simulink model "Model_14Bus_AC_DC_Microgrid"  (R2025a)
settings: Solver=ode23tb  StartTime=0.0  StopTime=0.1  MaxStep=1e-2  RelTol=1e-3
InitFcn:
  | Set_parameters_R2018
StopFcn:
  | Save_Data;
  | Graphics;
undefined symbols (not defined in the file): Clink, D1, Delta, dis1, dis10, dis11, dis12, dis13, dis14, dis2, dis3, dis4, dis5, dis6, dis7, dis8, dis9, Fc, Fnom, Hydride, Increment_MPPT, Ion, Ki_Ireg, Ki_VDCreg, Kp_Ireg, Kp_VDCreg, LimitL_Ireg, LimitL_VDCreg, Limits_MPPT, LimitU_Ireg, LimitU_VDCreg, Lithium, max_min, Metal, Nickel, P_Load_2, P_Load_3, Pnom, Pnom_T1, Pnom_T2, Pnom_T3, Pnom_xfo, Ql_Load_2, Ql_Load_3, R_Load_9, R_Load_DC, RL, Rl, RLff, Rls, sigbuilder_block, Ts, Ts_Control, Ts_Power, V1_LL_T3, Vf, Vfd, Vnom_dc, Vnom_DC, Vnom_Diesel ... (+5)
libraries: spsRMSLib x87, spsCurrentMeasurementLib x47, spsThreePhaseVIMeasurementLib x23, spsVoltageMeasurementLib x21, spsPowerLib x21, spsTHDLib x20, spsThreePhaseSeriesRLCBranchLib x20, spsSeriesRLCBranchLib x19, spsIGBTDiodeLib x14, spsThreePhaseBreakerLib x14, powerlib_extras x14, simulink x12
(part 5 of 9)

== system Model_14Bus_AC_DC_Microgrid/Boost -buck Bi-directional converter DC //CD 1 0.65 kW/ref ==
  note: 1 -charge
      | 0-discharge
  Constant2 : Constant  Value=max_min
  Constant3 : Constant  Value=max_min
  Current reference (battery charge) OP_Max : Constant  Value=5
  Current reference (battery discharge) OP_Max1 : Constant  Value=-5
  Min Demand OP_min : Constant  Value=3
  Min Demand OP_min1 : Constant  Value=-3
  Switch : Switch  Criteria=u2 > Threshold  SaturateOnIntegerOverflow=off  InputSameDT=off
  Switch1 : Switch  Criteria=u2 > Threshold  SaturateOnIntegerOverflow=off  InputSameDT=off
  Switch3 : Switch  Criteria=u2 > Threshold  SaturateOnIntegerOverflow=off  InputSameDT=off
  Vref1 : Constant
  ref : Outport  VectorParamsAs1DForOutWhenUnconnected=off
  wires:
  Constant3/1 -> Switch3/2
  Switch3/1 -> Switch/3
  Switch1/1 -> Switch/1
  Vref1/1 -> Switch/2
  Min Demand OP_min/1 -> Switch1/3
  Current reference (battery charge) OP_Max/1 -> Switch1/1
  Min Demand OP_min1/1 -> Switch3/3
  Constant2/1 -> Switch1/2
  Current reference (battery discharge) OP_Max1/1 -> Switch3/1
  Switch/1 -> ref/1

== system Model_14Bus_AC_DC_Microgrid/Boost converter DC //CD 2 5 kHz - 300V /  ==
  V_PV : Inport
  I_PV : Inport  Port=2
  Duty Cycle : Constant  Value=0.34
  PWM Generator (DC-DC) : spsPWMGeneratorDCDCLib/PWM Generator (DC-DC)  Fsw=fc  Ts=Ts_Power
  Terminator1 : Terminator
  Terminator2 : Terminator
  Pulses : Outport  VectorParamsAs1DForOutWhenUnconnected=off
  tag scope: D=global
  wires:
  V_PV/1 -> Terminator1/1
  I_PV/1 -> Terminator2/1
  PWM Generator (DC-DC)/1 -> Pulses/1
  Duty Cycle/1 -> [D], PWM Generator (DC-DC)/1

== system Model_14Bus_AC_DC_Microgrid/Bus_1/PLL ==
  Vabc_LN_pu : Inport
  2pi60'1 : Constant  Value=2*pi*60
  2pi60'2 : Constant  Value=2*pi*60
  2pi60'3 : Constant  Value=2*pi*60
  Constant : Constant  Value=90
  Demux : Demux  Outputs=3
  Gain1 : Gain  Gain=180/pi  SaturateOnIntegerOverflow=on  OutDataTypeStr=Inherit: Same as input  ParamDataTypeStr=Inherit: Same as input
  Gain2 : Gain  Gain=180/pi  SaturateOnIntegerOverflow=on  OutDataTypeStr=Inherit: Same as input  ParamDataTypeStr=Inherit: Same as input
  Gain3 : Gain  Gain=180/pi  SaturateOnIntegerOverflow=on  OutDataTypeStr=Inherit: Same as input  ParamDataTypeStr=Inherit: Same as input
  Mux : Mux  Inputs=3
  Pll1 : Subsystem
  Pll2 : Subsystem
  Pll3 : Subsystem
  Sum : Sum  Inputs=|++
  delta_abc : Outport  VectorParamsAs1DForOutWhenUnconnected=off
  wires:
  Vabc_LN_pu/1 -> Demux/1
  Demux/1 -> Pll3/1(señal)
  2pi60'3/1 -> Pll3/2(w)
  Pll3/1(f cos (rad)) -> Gain1/1
  Demux/2 -> Pll1/1(señal)
  2pi60'1/1 -> Pll1/2(w)
  Gain2/1 -> Mux/2
  Demux/3 -> Pll2/1(señal)
  2pi60'2/1 -> Pll2/2(w)
  Pll2/1(f cos (rad)) -> Gain3/1
  Gain3/1 -> Mux/3
  Pll1/1(f cos (rad)) -> Gain2/1
  Mux/1 -> Sum/1
  Gain1/1 -> Mux/1
  Constant/1 -> Sum/2
  Sum/1 -> delta_abc/1

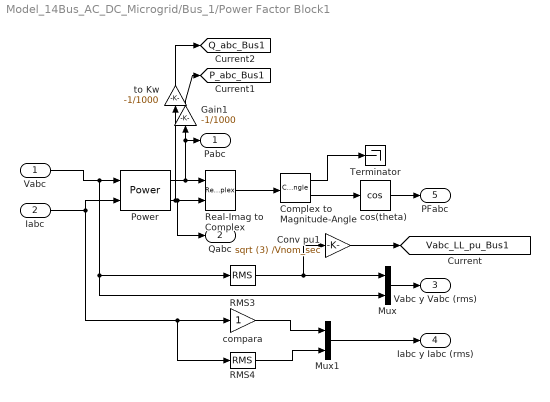
== system Model_14Bus_AC_DC_Microgrid/Bus_1/Power Factor Block1 ==
  Vabc : Inport
  Iabc : Inport  Port=2
  Complex to Magnitude-Angle : ComplexToMagnitudeAngle
  Conv pu1 : Gain  Gain=sqrt (3) /Vnom_sec  SaturateOnIntegerOverflow=on  OutDataTypeStr=Inherit: Same as input  ParamDataTypeStr=Inherit: Same as input
  Gain1 : Gain  Gain=-1/1000
  Mux : Mux  Inputs=2
  Mux1 : Mux  Inputs=2
  Power : spsPowerLib/Power  Freq=Freq  Vinit=Vinit  Iinit=Iinit  Ts=Ts
  RMS3 : spsRMSLib/RMS  TrueRMS=on  Freq=60  RMSInit=0  Ts=0
  RMS4 : spsRMSLib/RMS  TrueRMS=on  Freq=60  RMSInit=0  Ts=0
  Real-Imag to Complex : RealImagToComplex
  Terminator : Terminator
  compara : Gain  SaturateOnIntegerOverflow=on  OutDataTypeStr=Inherit: Same as input  ParamDataTypeStr=Inherit: Same as input
  cos(theta) : Trigonometry  Operator=cos
  to Kw : Gain  Gain=-1/1000
  Pabc : Outport  VectorParamsAs1DForOutWhenUnconnected=off
  Qabc : Outport  Port=2  VectorParamsAs1DForOutWhenUnconnected=off
  Vabc y Vabc (rms) : Outport  Port=3  VectorParamsAs1DForOutWhenUnconnected=off
  Iabc y Iabc (rms) : Outport  Port=4  VectorParamsAs1DForOutWhenUnconnected=off
  "PFabc " : Outport  Port=5  VectorParamsAs1DForOutWhenUnconnected=off
  tag scope: P_abc_Bus1=global, Q_abc_Bus1=global, Vabc_LL_pu_Bus1=global
  wires:
  Power/1 -> Gain1/1, Pabc/1, Real-Imag to Complex/1
  Power/2 -> Qabc/1, Real-Imag to Complex/2, to Kw/1
  Complex to Magnitude-Angle/2 -> cos(theta)/1
  Real-Imag to Complex/1 -> Complex to Magnitude-Angle/1
  cos(theta)/1 -> "PFabc "/1
  Complex to Magnitude-Angle/1 -> Terminator/1
  Iabc/1 -> RMS4/1, compara/1, Power/2
  RMS4/1 -> Mux1/2
  Mux1/1 -> Iabc y Iabc (rms)/1
  Mux/1 -> Vabc y Vabc (rms)/1
  Vabc/1 -> Power/1, Mux/2, RMS3/1
  compara/1 -> Mux1/1
  RMS3/1 -> Conv pu1/1, Mux/1
  Conv pu1/1 -> [Vabc_LL_pu_Bus1]
  to Kw/1 -> [Q_abc_Bus1]
  Gain1/1 -> [P_abc_Bus1]

== system Model_14Bus_AC_DC_Microgrid/Bus_10/PLL ==
  Vabc_LN_pu : Inport
  2pi60'1 : Constant  Value=2*pi*60
  2pi60'2 : Constant  Value=2*pi*60
  2pi60'3 : Constant  Value=2*pi*60
  Constant : Constant  Value=90
  Demux : Demux  Outputs=3
  Gain1 : Gain  Gain=180/pi  SaturateOnIntegerOverflow=on  OutDataTypeStr=Inherit: Same as input  ParamDataTypeStr=Inherit: Same as input
  Gain2 : Gain  Gain=180/pi  SaturateOnIntegerOverflow=on  OutDataTypeStr=Inherit: Same as input  ParamDataTypeStr=Inherit: Same as input
  Gain3 : Gain  Gain=180/pi  SaturateOnIntegerOverflow=on  OutDataTypeStr=Inherit: Same as input  ParamDataTypeStr=Inherit: Same as input
  Mux : Mux  Inputs=3
  Pll1 : Subsystem
  Pll2 : Subsystem
  Pll3 : Subsystem
  Sum : Sum  Inputs=|++
  delta_abc : Outport  VectorParamsAs1DForOutWhenUnconnected=off
  wires:
  Vabc_LN_pu/1 -> Demux/1
  Demux/1 -> Pll3/1(señal)
  2pi60'3/1 -> Pll3/2(w)
  Pll3/1(f cos (rad)) -> Gain1/1
  Demux/2 -> Pll1/1(señal)
  2pi60'1/1 -> Pll1/2(w)
  Gain2/1 -> Mux/2
  Demux/3 -> Pll2/1(señal)
  2pi60'2/1 -> Pll2/2(w)
  Pll2/1(f cos (rad)) -> Gain3/1
  Gain3/1 -> Mux/3
  Pll1/1(f cos (rad)) -> Gain2/1
  Mux/1 -> Sum/1
  Gain1/1 -> Mux/1
  Constant/1 -> Sum/2
  Sum/1 -> delta_abc/1

== system Model_14Bus_AC_DC_Microgrid/Bus_10/Power Factor Block1 ==
  Vabc : Inport
  Iabc : Inport  Port=2
  Complex to Magnitude-Angle : ComplexToMagnitudeAngle
  Conv pu2 : Gain  Gain=sqrt (3) /Vnom_prim  SaturateOnIntegerOverflow=on  OutDataTypeStr=Inherit: Same as input  ParamDataTypeStr=Inherit: Same as input
  Mux : Mux  Inputs=2
  Mux1 : Mux  Inputs=2
  Power : spsPowerLib/Power  Freq=Freq  Vinit=Vinit  Iinit=Iinit  Ts=Ts
  RMS3 : spsRMSLib/RMS  TrueRMS=on  Freq=60  RMSInit=0  Ts=0
  RMS4 : spsRMSLib/RMS  TrueRMS=on  Freq=60  RMSInit=0  Ts=0
  Real-Imag to Complex : RealImagToComplex
  Terminator : Terminator
  compara : Gain  SaturateOnIntegerOverflow=on  OutDataTypeStr=Inherit: Same as input  ParamDataTypeStr=Inherit: Same as input
  cos(theta) : Trigonometry  Operator=cos
  to Kw : Gain  Gain=1/1000
  to Kw1 : Gain  Gain=1/1000
  Pabc : Outport  VectorParamsAs1DForOutWhenUnconnected=off
  Qabc : Outport  Port=2  VectorParamsAs1DForOutWhenUnconnected=off
  Vabc y Vabc (rms) : Outport  Port=3  VectorParamsAs1DForOutWhenUnconnected=off
  Iabc y Iabc (rms) : Outport  Port=4  VectorParamsAs1DForOutWhenUnconnected=off
  "PFabc " : Outport  Port=5  VectorParamsAs1DForOutWhenUnconnected=off
  tag scope: P_abc_Bus10=global, Q_abc_Bus10=global, Vabc_LL_pu_Bus10=global
  wires:
  Complex to Magnitude-Angle/2 -> cos(theta)/1
  Real-Imag to Complex/1 -> Complex to Magnitude-Angle/1
  cos(theta)/1 -> "PFabc "/1
  Complex to Magnitude-Angle/1 -> Terminator/1
  Iabc/1 -> RMS4/1, compara/1, Power/2
  RMS4/1 -> Mux1/2
  Mux1/1 -> Iabc y Iabc (rms)/1
  Mux/1 -> Vabc y Vabc (rms)/1
  Vabc/1 -> Power/1, Mux/2, RMS3/1
  compara/1 -> Mux1/1
  Conv pu2/1 -> [Vabc_LL_pu_Bus10]
  RMS3/1 -> Conv pu2/1, Mux/1
  Power/1 -> to Kw1/1, Pabc/1, Real-Imag to Complex/1
  Power/2 -> Qabc/1, Real-Imag to Complex/2, to Kw/1
  to Kw/1 -> [Q_abc_Bus10]
  to Kw1/1 -> [P_abc_Bus10]

== system Model_14Bus_AC_DC_Microgrid/Bus_11/PLL ==
  Vabc_LN_pu : Inport
  2pi60'1 : Constant  Value=2*pi*60
  2pi60'2 : Constant  Value=2*pi*60
  2pi60'3 : Constant  Value=2*pi*60
  Constant : Constant  Value=90
  Demux : Demux  Outputs=3
  Gain1 : Gain  Gain=180/pi  SaturateOnIntegerOverflow=on  OutDataTypeStr=Inherit: Same as input  ParamDataTypeStr=Inherit: Same as input
  Gain2 : Gain  Gain=180/pi  SaturateOnIntegerOverflow=on  OutDataTypeStr=Inherit: Same as input  ParamDataTypeStr=Inherit: Same as input
  Gain3 : Gain  Gain=180/pi  SaturateOnIntegerOverflow=on  OutDataTypeStr=Inherit: Same as input  ParamDataTypeStr=Inherit: Same as input
  Mux : Mux  Inputs=3
  Pll1 : Subsystem
  Pll2 : Subsystem
  Pll3 : Subsystem
  Sum : Sum  Inputs=|++
  delta_abc : Outport  VectorParamsAs1DForOutWhenUnconnected=off
  wires:
  Vabc_LN_pu/1 -> Demux/1
  Demux/1 -> Pll3/1(señal)
  2pi60'3/1 -> Pll3/2(w)
  Pll3/1(f cos (rad)) -> Gain1/1
  Demux/2 -> Pll1/1(señal)
  2pi60'1/1 -> Pll1/2(w)
  Gain2/1 -> Mux/2
  Demux/3 -> Pll2/1(señal)
  2pi60'2/1 -> Pll2/2(w)
  Pll2/1(f cos (rad)) -> Gain3/1
  Gain3/1 -> Mux/3
  Pll1/1(f cos (rad)) -> Gain2/1
  Mux/1 -> Sum/1
  Gain1/1 -> Mux/1
  Constant/1 -> Sum/2
  Sum/1 -> delta_abc/1

== system Model_14Bus_AC_DC_Microgrid/Bus_11/Power Factor Block1 ==
  Vabc : Inport
  Iabc : Inport  Port=2
  Complex to Magnitude-Angle : ComplexToMagnitudeAngle
  Conv pu2 : Gain  Gain=sqrt (3) /Vnom_prim  SaturateOnIntegerOverflow=on  OutDataTypeStr=Inherit: Same as input  ParamDataTypeStr=Inherit: Same as input
  Mux : Mux  Inputs=2
  Mux1 : Mux  Inputs=2
  Power : spsPowerLib/Power  Freq=Freq  Vinit=Vinit  Iinit=Iinit  Ts=Ts
  RMS3 : spsRMSLib/RMS  TrueRMS=on  Freq=60  RMSInit=0  Ts=0
  RMS4 : spsRMSLib/RMS  TrueRMS=on  Freq=60  RMSInit=0  Ts=0
  Real-Imag to Complex : RealImagToComplex
  Terminator : Terminator
  compara : Gain  SaturateOnIntegerOverflow=on  OutDataTypeStr=Inherit: Same as input  ParamDataTypeStr=Inherit: Same as input
  cos(theta) : Trigonometry  Operator=cos
  to Kw : Gain  Gain=1/1000
  to Kw1 : Gain  Gain=1/1000
  Pabc : Outport  VectorParamsAs1DForOutWhenUnconnected=off
  Qabc : Outport  Port=2  VectorParamsAs1DForOutWhenUnconnected=off
  Vabc y Vabc (rms) : Outport  Port=3  VectorParamsAs1DForOutWhenUnconnected=off
  Iabc y Iabc (rms) : Outport  Port=4  VectorParamsAs1DForOutWhenUnconnected=off
  "PFabc " : Outport  Port=5  VectorParamsAs1DForOutWhenUnconnected=off
  tag scope: P_abc_Bus11=global, Q_abc_Bus11=global, Vabc_LL_pu_Bus11=global
  wires:
  Complex to Magnitude-Angle/2 -> cos(theta)/1
  Real-Imag to Complex/1 -> Complex to Magnitude-Angle/1
  cos(theta)/1 -> "PFabc "/1
  Complex to Magnitude-Angle/1 -> Terminator/1
  Iabc/1 -> RMS4/1, compara/1, Power/2
  RMS4/1 -> Mux1/2
  Mux1/1 -> Iabc y Iabc (rms)/1
  Mux/1 -> Vabc y Vabc (rms)/1
  Vabc/1 -> Power/1, Mux/2, RMS3/1
  compara/1 -> Mux1/1
  RMS3/1 -> Conv pu2/1, Mux/1
  Conv pu2/1 -> [Vabc_LL_pu_Bus11]
  Power/2 -> Qabc/1, Real-Imag to Complex/2, to Kw/1
  Power/1 -> to Kw1/1, Pabc/1, Real-Imag to Complex/1
  to Kw/1 -> [Q_abc_Bus11]
  to Kw1/1 -> [P_abc_Bus11]

== system Model_14Bus_AC_DC_Microgrid/Bus_12/PLL ==
  Vabc_LN_pu : Inport
  2pi60'1 : Constant  Value=2*pi*60
  2pi60'2 : Constant  Value=2*pi*60
  2pi60'3 : Constant  Value=2*pi*60
  Constant : Constant  Value=90
  Demux : Demux  Outputs=3
  Gain1 : Gain  Gain=180/pi  SaturateOnIntegerOverflow=on  OutDataTypeStr=Inherit: Same as input  ParamDataTypeStr=Inherit: Same as input
  Gain2 : Gain  Gain=180/pi  SaturateOnIntegerOverflow=on  OutDataTypeStr=Inherit: Same as input  ParamDataTypeStr=Inherit: Same as input
  Gain3 : Gain  Gain=180/pi  SaturateOnIntegerOverflow=on  OutDataTypeStr=Inherit: Same as input  ParamDataTypeStr=Inherit: Same as input
  Mux : Mux  Inputs=3
  Pll1 : Subsystem
  Pll2 : Subsystem
  Pll3 : Subsystem
  Sum : Sum  Inputs=|++
  delta_abc : Outport  VectorParamsAs1DForOutWhenUnconnected=off
  wires:
  Vabc_LN_pu/1 -> Demux/1
  Demux/1 -> Pll3/1(señal)
  2pi60'3/1 -> Pll3/2(w)
  Pll3/1(f cos (rad)) -> Gain1/1
  Demux/2 -> Pll1/1(señal)
  2pi60'1/1 -> Pll1/2(w)
  Gain2/1 -> Mux/2
  Demux/3 -> Pll2/1(señal)
  2pi60'2/1 -> Pll2/2(w)
  Pll2/1(f cos (rad)) -> Gain3/1
  Gain3/1 -> Mux/3
  Pll1/1(f cos (rad)) -> Gain2/1
  Mux/1 -> Sum/1
  Gain1/1 -> Mux/1
  Constant/1 -> Sum/2
  Sum/1 -> delta_abc/1

== system Model_14Bus_AC_DC_Microgrid/Bus_12/Power Factor Block1 ==
  Vabc : Inport
  Iabc : Inport  Port=2
  Complex to Magnitude-Angle : ComplexToMagnitudeAngle
  Conv pu2 : Gain  Gain=sqrt (3) /Vnom_prim  SaturateOnIntegerOverflow=on  OutDataTypeStr=Inherit: Same as input  ParamDataTypeStr=Inherit: Same as input
  Mux : Mux  Inputs=2
  Mux1 : Mux  Inputs=2
  Power : spsPowerLib/Power  Freq=Freq  Vinit=Vinit  Iinit=Iinit  Ts=Ts
  RMS3 : spsRMSLib/RMS  TrueRMS=on  Freq=60  RMSInit=0  Ts=0
  RMS4 : spsRMSLib/RMS  TrueRMS=on  Freq=60  RMSInit=0  Ts=0
  Real-Imag to Complex : RealImagToComplex
  Terminator : Terminator
  compara : Gain  SaturateOnIntegerOverflow=on  OutDataTypeStr=Inherit: Same as input  ParamDataTypeStr=Inherit: Same as input
  cos(theta) : Trigonometry  Operator=cos
  to Kw : Gain  Gain=1/1000
  to Kw1 : Gain  Gain=1/1000
  Pabc : Outport  VectorParamsAs1DForOutWhenUnconnected=off
  Qabc : Outport  Port=2  VectorParamsAs1DForOutWhenUnconnected=off
  Vabc y Vabc (rms) : Outport  Port=3  VectorParamsAs1DForOutWhenUnconnected=off
  Iabc y Iabc (rms) : Outport  Port=4  VectorParamsAs1DForOutWhenUnconnected=off
  "PFabc " : Outport  Port=5  VectorParamsAs1DForOutWhenUnconnected=off
  tag scope: P_abc_Bus12=global, Q_abc_Bus12=global, Vabc_LL_pu_Bus12=global
  wires:
  Complex to Magnitude-Angle/2 -> cos(theta)/1
  Real-Imag to Complex/1 -> Complex to Magnitude-Angle/1
  cos(theta)/1 -> "PFabc "/1
  Complex to Magnitude-Angle/1 -> Terminator/1
  Iabc/1 -> RMS4/1, compara/1, Power/2
  RMS4/1 -> Mux1/2
  Mux1/1 -> Iabc y Iabc (rms)/1
  Mux/1 -> Vabc y Vabc (rms)/1
  Vabc/1 -> Power/1, Mux/2, RMS3/1
  compara/1 -> Mux1/1
  RMS3/1 -> Conv pu2/1, Mux/1
  Conv pu2/1 -> [Vabc_LL_pu_Bus12]
  Power/1 -> to Kw/1, Pabc/1, Real-Imag to Complex/1
  Power/2 -> to Kw1/1, Qabc/1, Real-Imag to Complex/2
  to Kw1/1 -> [Q_abc_Bus12]
  to Kw/1 -> [P_abc_Bus12]

== system Model_14Bus_AC_DC_Microgrid/Bus_14 /PLL ==
  Vabc_LN_pu : Inport
  2pi60'1 : Constant  Value=2*pi*60
  2pi60'2 : Constant  Value=2*pi*60
  2pi60'3 : Constant  Value=2*pi*60
  Constant : Constant  Value=90
  Demux : Demux  Outputs=3
  Gain1 : Gain  Gain=180/pi  SaturateOnIntegerOverflow=on  OutDataTypeStr=Inherit: Same as input  ParamDataTypeStr=Inherit: Same as input
  Gain2 : Gain  Gain=180/pi  SaturateOnIntegerOverflow=on  OutDataTypeStr=Inherit: Same as input  ParamDataTypeStr=Inherit: Same as input
  Gain3 : Gain  Gain=180/pi  SaturateOnIntegerOverflow=on  OutDataTypeStr=Inherit: Same as input  ParamDataTypeStr=Inherit: Same as input
  Mux : Mux  Inputs=3
  Pll1 : Subsystem
  Pll2 : Subsystem
  Pll3 : Subsystem
  Sum : Sum  Inputs=|++
  delta_abc : Outport  VectorParamsAs1DForOutWhenUnconnected=off
  wires:
  Vabc_LN_pu/1 -> Demux/1
  Demux/1 -> Pll3/1(señal)
  2pi60'3/1 -> Pll3/2(w)
  Pll3/1(f cos (rad)) -> Gain1/1
  Demux/2 -> Pll1/1(señal)
  2pi60'1/1 -> Pll1/2(w)
  Gain2/1 -> Mux/2
  Demux/3 -> Pll2/1(señal)
  2pi60'2/1 -> Pll2/2(w)
  Pll2/1(f cos (rad)) -> Gain3/1
  Gain3/1 -> Mux/3
  Pll1/1(f cos (rad)) -> Gain2/1
  Mux/1 -> Sum/1
  Gain1/1 -> Mux/1
  Constant/1 -> Sum/2
  Sum/1 -> delta_abc/1

== system Model_14Bus_AC_DC_Microgrid/Bus_14 /Power Factor Block1 ==
  Vabc : Inport
  Iabc : Inport  Port=2
  Complex to Magnitude-Angle : ComplexToMagnitudeAngle
  Conv pu2 : Gain  Gain=sqrt (3) /Vnom_prim  SaturateOnIntegerOverflow=on  OutDataTypeStr=Inherit: Same as input  ParamDataTypeStr=Inherit: Same as input
  Mux : Mux  Inputs=2
  Mux1 : Mux  Inputs=2
  Power : spsPowerLib/Power  Freq=Freq  Vinit=Vinit  Iinit=Iinit  Ts=Ts
  RMS3 : spsRMSLib/RMS  TrueRMS=on  Freq=60  RMSInit=0  Ts=0
  RMS4 : spsRMSLib/RMS  TrueRMS=on  Freq=60  RMSInit=0  Ts=0
  Real-Imag to Complex : RealImagToComplex
  Terminator : Terminator
  compara : Gain  SaturateOnIntegerOverflow=on  OutDataTypeStr=Inherit: Same as input  ParamDataTypeStr=Inherit: Same as input
  cos(theta) : Trigonometry  Operator=cos
  to Kw : Gain  Gain=1/1000
  to Kw1 : Gain  Gain=1/1000
  Pabc : Outport  VectorParamsAs1DForOutWhenUnconnected=off
  Qabc : Outport  Port=2  VectorParamsAs1DForOutWhenUnconnected=off
  Vabc y Vabc (rms) : Outport  Port=3  VectorParamsAs1DForOutWhenUnconnected=off
  Iabc y Iabc (rms) : Outport  Port=4  VectorParamsAs1DForOutWhenUnconnected=off
  "PFabc " : Outport  Port=5  VectorParamsAs1DForOutWhenUnconnected=off
  tag scope: P_abc_Bus14=global, Q_abc_Bus14=global, Vabc_LL_pu_Bus14=global
  wires:
  Complex to Magnitude-Angle/2 -> cos(theta)/1
  Real-Imag to Complex/1 -> Complex to Magnitude-Angle/1
  cos(theta)/1 -> "PFabc "/1
  Complex to Magnitude-Angle/1 -> Terminator/1
  Iabc/1 -> RMS4/1, compara/1, Power/2
  RMS4/1 -> Mux1/2
  Mux1/1 -> Iabc y Iabc (rms)/1
  Mux/1 -> Vabc y Vabc (rms)/1
  Vabc/1 -> Power/1, Mux/2, RMS3/1
  compara/1 -> Mux1/1
  RMS3/1 -> Conv pu2/1, Mux/1
  Conv pu2/1 -> [Vabc_LL_pu_Bus14]
  Power/2 -> Qabc/1, Real-Imag to Complex/2, to Kw1/1
  Power/1 -> to Kw/1, Pabc/1, Real-Imag to Complex/1
  to Kw1/1 -> [Q_abc_Bus14]
  to Kw/1 -> [P_abc_Bus14]

== system Model_14Bus_AC_DC_Microgrid/Bus_2/PLL ==
  Vabc_LN_pu : Inport
  2pi60'1 : Constant  Value=2*pi*60
  2pi60'2 : Constant  Value=2*pi*60
  2pi60'3 : Constant  Value=2*pi*60
  Constant : Constant  Value=90
  Demux : Demux  Outputs=3
  Gain1 : Gain  Gain=180/pi  SaturateOnIntegerOverflow=on  OutDataTypeStr=Inherit: Same as input  ParamDataTypeStr=Inherit: Same as input
  Gain2 : Gain  Gain=180/pi  SaturateOnIntegerOverflow=on  OutDataTypeStr=Inherit: Same as input  ParamDataTypeStr=Inherit: Same as input
  Gain3 : Gain  Gain=180/pi  SaturateOnIntegerOverflow=on  OutDataTypeStr=Inherit: Same as input  ParamDataTypeStr=Inherit: Same as input
  Mux : Mux  Inputs=3
  Pll1 : Subsystem
  Pll2 : Subsystem
  Pll3 : Subsystem
  Sum : Sum  Inputs=|++
  delta_abc : Outport  VectorParamsAs1DForOutWhenUnconnected=off
  wires:
  Vabc_LN_pu/1 -> Demux/1
  Demux/1 -> Pll3/1(señal)
  2pi60'3/1 -> Pll3/2(w)
  Pll3/1(f cos (rad)) -> Gain1/1
  Demux/2 -> Pll1/1(señal)
  2pi60'1/1 -> Pll1/2(w)
  Gain2/1 -> Mux/2
  Demux/3 -> Pll2/1(señal)
  2pi60'2/1 -> Pll2/2(w)
  Pll2/1(f cos (rad)) -> Gain3/1
  Gain3/1 -> Mux/3
  Pll1/1(f cos (rad)) -> Gain2/1
  Mux/1 -> Sum/1
  Gain1/1 -> Mux/1
  Constant/1 -> Sum/2
  Sum/1 -> delta_abc/1

== system Model_14Bus_AC_DC_Microgrid/Bus_2/Power Factor Block1 ==
  Vabc : Inport
  Iabc : Inport  Port=2
  Complex to Magnitude-Angle : ComplexToMagnitudeAngle
  Conv pu1 : Gain  Gain=sqrt (3) /Vnom_sec  SaturateOnIntegerOverflow=on  OutDataTypeStr=Inherit: Same as input  ParamDataTypeStr=Inherit: Same as input
  Mux : Mux  Inputs=2
  Mux1 : Mux  Inputs=2
  Power : spsPowerLib/Power  Freq=Freq  Vinit=Vinit  Iinit=Iinit  Ts=Ts
  RMS3 : spsRMSLib/RMS  TrueRMS=on  Freq=60  RMSInit=0  Ts=0
  RMS4 : spsRMSLib/RMS  TrueRMS=on  Freq=60  RMSInit=0  Ts=0
  Real-Imag to Complex : RealImagToComplex
  Terminator : Terminator
  compara : Gain  SaturateOnIntegerOverflow=on  OutDataTypeStr=Inherit: Same as input  ParamDataTypeStr=Inherit: Same as input
  cos(theta) : Trigonometry  Operator=cos
  to Kw : Gain  Gain=-1/1000
  to Kw1 : Gain  Gain=-1/1000
  Pabc : Outport  VectorParamsAs1DForOutWhenUnconnected=off
  Qabc : Outport  Port=2  VectorParamsAs1DForOutWhenUnconnected=off
  Vabc y Vabc (rms) : Outport  Port=3  VectorParamsAs1DForOutWhenUnconnected=off
  Iabc y Iabc (rms) : Outport  Port=4  VectorParamsAs1DForOutWhenUnconnected=off
  "PFabc " : Outport  Port=5  VectorParamsAs1DForOutWhenUnconnected=off
  tag scope: P_abc_Bus2=global, Q_abc_Bus2=global, Vabc_LL_pu_Bus2=global
  wires:
  Complex to Magnitude-Angle/2 -> cos(theta)/1
  Real-Imag to Complex/1 -> Complex to Magnitude-Angle/1
  cos(theta)/1 -> "PFabc "/1
  Complex to Magnitude-Angle/1 -> Terminator/1
  Iabc/1 -> RMS4/1, compara/1, Power/2
  RMS4/1 -> Mux1/2
  Mux1/1 -> Iabc y Iabc (rms)/1
  Mux/1 -> Vabc y Vabc (rms)/1
  Vabc/1 -> Power/1, Mux/2, RMS3/1
  compara/1 -> Mux1/1
  RMS3/1 -> Conv pu1/1, Mux/1
  Conv pu1/1 -> [Vabc_LL_pu_Bus2]
  Power/1 -> to Kw1/1, Pabc/1, Real-Imag to Complex/1
  Power/2 -> to Kw/1, Qabc/1, Real-Imag to Complex/2
  to Kw/1 -> [Q_abc_Bus2]
  to Kw1/1 -> [P_abc_Bus2]

== system Model_14Bus_AC_DC_Microgrid/Bus_3/PLL ==
  Vabc_LN_pu : Inport
  2pi60'1 : Constant  Value=2*pi*60
  2pi60'2 : Constant  Value=2*pi*60
  2pi60'3 : Constant  Value=2*pi*60
  Constant : Constant  Value=90
  Demux : Demux  Outputs=3
  Gain1 : Gain  Gain=180/pi  SaturateOnIntegerOverflow=on  OutDataTypeStr=Inherit: Same as input  ParamDataTypeStr=Inherit: Same as input
  Gain2 : Gain  Gain=180/pi  SaturateOnIntegerOverflow=on  OutDataTypeStr=Inherit: Same as input  ParamDataTypeStr=Inherit: Same as input
  Gain3 : Gain  Gain=180/pi  SaturateOnIntegerOverflow=on  OutDataTypeStr=Inherit: Same as input  ParamDataTypeStr=Inherit: Same as input
  Mux : Mux  Inputs=3
  Pll1 : Subsystem
  Pll2 : Subsystem
  Pll3 : Subsystem
  Sum : Sum  Inputs=|++
  delta_abc : Outport  VectorParamsAs1DForOutWhenUnconnected=off
  wires:
  Vabc_LN_pu/1 -> Demux/1
  Demux/1 -> Pll3/1(señal)
  2pi60'3/1 -> Pll3/2(w)
  Pll3/1(f cos (rad)) -> Gain1/1
  Demux/2 -> Pll1/1(señal)
  2pi60'1/1 -> Pll1/2(w)
  Gain2/1 -> Mux/2
  Demux/3 -> Pll2/1(señal)
  2pi60'2/1 -> Pll2/2(w)
  Pll2/1(f cos (rad)) -> Gain3/1
  Gain3/1 -> Mux/3
  Pll1/1(f cos (rad)) -> Gain2/1
  Mux/1 -> Sum/1
  Gain1/1 -> Mux/1
  Constant/1 -> Sum/2
  Sum/1 -> delta_abc/1

== system Model_14Bus_AC_DC_Microgrid/Bus_3/Power Factor Block1 ==
  Vabc : Inport
  Iabc : Inport  Port=2
  Complex to Magnitude-Angle : ComplexToMagnitudeAngle
  Conv pu1 : Gain  Gain=sqrt (3) /Vnom_sec  SaturateOnIntegerOverflow=on  OutDataTypeStr=Inherit: Same as input  ParamDataTypeStr=Inherit: Same as input
  Mux : Mux  Inputs=2
  Mux1 : Mux  Inputs=2
  Power : spsPowerLib/Power  Freq=Freq  Vinit=Vinit  Iinit=Iinit  Ts=Ts
  RMS3 : spsRMSLib/RMS  TrueRMS=on  Freq=60  RMSInit=0  Ts=0
  RMS4 : spsRMSLib/RMS  TrueRMS=on  Freq=60  RMSInit=0  Ts=0
  Real-Imag to Complex : RealImagToComplex
  Terminator : Terminator
  compara : Gain  SaturateOnIntegerOverflow=on  OutDataTypeStr=Inherit: Same as input  ParamDataTypeStr=Inherit: Same as input
  cos(theta) : Trigonometry  Operator=cos
  to Kw : Gain  Gain=1/1000
  to Kw1 : Gain  Gain=1/1000
  Pabc : Outport  VectorParamsAs1DForOutWhenUnconnected=off
  Qabc : Outport  Port=2  VectorParamsAs1DForOutWhenUnconnected=off
  Vabc y Vabc (rms) : Outport  Port=3  VectorParamsAs1DForOutWhenUnconnected=off
  Iabc y Iabc (rms) : Outport  Port=4  VectorParamsAs1DForOutWhenUnconnected=off
  "PFabc " : Outport  Port=5  VectorParamsAs1DForOutWhenUnconnected=off
  tag scope: P_abc_Bus3=global, Q_abc_Bus3=global, Vabc_LL_pu_Bus3=global
  wires:
  Complex to Magnitude-Angle/2 -> cos(theta)/1
  Real-Imag to Complex/1 -> Complex to Magnitude-Angle/1
  cos(theta)/1 -> "PFabc "/1
  Complex to Magnitude-Angle/1 -> Terminator/1
  Iabc/1 -> RMS4/1, compara/1, Power/2
  RMS4/1 -> Mux1/2
  Mux1/1 -> Iabc y Iabc (rms)/1
  Mux/1 -> Vabc y Vabc (rms)/1
  Vabc/1 -> Power/1, Mux/2, RMS3/1
  compara/1 -> Mux1/1
  Conv pu1/1 -> [Vabc_LL_pu_Bus3]
  RMS3/1 -> Conv pu1/1, Mux/1
  Power/2 -> Qabc/1, Real-Imag to Complex/2, to Kw/1
  Power/1 -> to Kw1/1, Pabc/1, Real-Imag to Complex/1
  to Kw/1 -> [Q_abc_Bus3]
  to Kw1/1 -> [P_abc_Bus3]

== system Model_14Bus_AC_DC_Microgrid/Bus_4/PLL ==
  Vabc_LN_pu : Inport
  2pi60'1 : Constant  Value=2*pi*60
  2pi60'2 : Constant  Value=2*pi*60
  2pi60'3 : Constant  Value=2*pi*60
  Constant : Constant  Value=90
  Demux : Demux  Outputs=3
  Gain1 : Gain  Gain=180/pi  SaturateOnIntegerOverflow=on  OutDataTypeStr=Inherit: Same as input  ParamDataTypeStr=Inherit: Same as input
  Gain2 : Gain  Gain=180/pi  SaturateOnIntegerOverflow=on  OutDataTypeStr=Inherit: Same as input  ParamDataTypeStr=Inherit: Same as input
  Gain3 : Gain  Gain=180/pi  SaturateOnIntegerOverflow=on  OutDataTypeStr=Inherit: Same as input  ParamDataTypeStr=Inherit: Same as input
  Mux : Mux  Inputs=3
  Pll1 : Subsystem
  Pll2 : Subsystem
  Pll3 : Subsystem
  Sum : Sum  Inputs=|++
  delta_abc : Outport  VectorParamsAs1DForOutWhenUnconnected=off
  wires:
  Vabc_LN_pu/1 -> Demux/1
  Demux/1 -> Pll3/1(señal)
  2pi60'3/1 -> Pll3/2(w)
  Pll3/1(f cos (rad)) -> Gain1/1
  Demux/2 -> Pll1/1(señal)
  2pi60'1/1 -> Pll1/2(w)
  Gain2/1 -> Mux/2
  Demux/3 -> Pll2/1(señal)
  2pi60'2/1 -> Pll2/2(w)
  Pll2/1(f cos (rad)) -> Gain3/1
  Gain3/1 -> Mux/3
  Pll1/1(f cos (rad)) -> Gain2/1
  Mux/1 -> Sum/1
  Gain1/1 -> Mux/1
  Constant/1 -> Sum/2
  Sum/1 -> delta_abc/1

== system Model_14Bus_AC_DC_Microgrid/Bus_4/Power Factor Block1 ==
  Vabc : Inport
  Iabc : Inport  Port=2
  Complex to Magnitude-Angle : ComplexToMagnitudeAngle
  Conv pu1 : Gain  Gain=sqrt (3) /Vnom_sec  SaturateOnIntegerOverflow=on  OutDataTypeStr=Inherit: Same as input  ParamDataTypeStr=Inherit: Same as input
  Mux : Mux  Inputs=2
  Mux1 : Mux  Inputs=2
  Power : spsPowerLib/Power  Freq=Freq  Vinit=Vinit  Iinit=Iinit  Ts=Ts
  RMS3 : spsRMSLib/RMS  TrueRMS=on  Freq=60  RMSInit=0  Ts=0
  RMS4 : spsRMSLib/RMS  TrueRMS=on  Freq=60  RMSInit=0  Ts=0
  Real-Imag to Complex : RealImagToComplex
  Terminator : Terminator
  compara : Gain  SaturateOnIntegerOverflow=on  OutDataTypeStr=Inherit: Same as input  ParamDataTypeStr=Inherit: Same as input
  cos(theta) : Trigonometry  Operator=cos
  to Kw : Gain  Gain=1/1000
  to Kw1 : Gain  Gain=1/1000
  Pabc : Outport  VectorParamsAs1DForOutWhenUnconnected=off
  Qabc : Outport  Port=2  VectorParamsAs1DForOutWhenUnconnected=off
  Vabc y Vabc (rms) : Outport  Port=3  VectorParamsAs1DForOutWhenUnconnected=off
  Iabc y Iabc (rms) : Outport  Port=4  VectorParamsAs1DForOutWhenUnconnected=off
  "PFabc " : Outport  Port=5  VectorParamsAs1DForOutWhenUnconnected=off
  tag scope: P_abc_Bus4=global, Q_abc_Bus4=global, Vabc_LL_pu_Bus4=global
  wires:
  Complex to Magnitude-Angle/2 -> cos(theta)/1
  Real-Imag to Complex/1 -> Complex to Magnitude-Angle/1
  cos(theta)/1 -> "PFabc "/1
  Complex to Magnitude-Angle/1 -> Terminator/1
  Iabc/1 -> RMS4/1, compara/1, Power/2
  RMS4/1 -> Mux1/2
  Mux1/1 -> Iabc y Iabc (rms)/1
  Mux/1 -> Vabc y Vabc (rms)/1
  Vabc/1 -> Power/1, Mux/2, RMS3/1
  compara/1 -> Mux1/1
  Conv pu1/1 -> [Vabc_LL_pu_Bus4]
  RMS3/1 -> Conv pu1/1, Mux/1
  Power/2 -> Qabc/1, Real-Imag to Complex/2, to Kw/1
  Power/1 -> to Kw1/1, Pabc/1, Real-Imag to Complex/1
  to Kw/1 -> [Q_abc_Bus4]
  to Kw1/1 -> [P_abc_Bus4]

== system Model_14Bus_AC_DC_Microgrid/Bus_5/PLL ==
  Vabc_LN_pu : Inport
  2pi60'1 : Constant  Value=2*pi*60
  2pi60'2 : Constant  Value=2*pi*60
  2pi60'3 : Constant  Value=2*pi*60
  Constant : Constant  Value=90
  Demux : Demux  Outputs=3
  Gain1 : Gain  Gain=180/pi  SaturateOnIntegerOverflow=on  OutDataTypeStr=Inherit: Same as input  ParamDataTypeStr=Inherit: Same as input
  Gain2 : Gain  Gain=180/pi  SaturateOnIntegerOverflow=on  OutDataTypeStr=Inherit: Same as input  ParamDataTypeStr=Inherit: Same as input
  Gain3 : Gain  Gain=180/pi  SaturateOnIntegerOverflow=on  OutDataTypeStr=Inherit: Same as input  ParamDataTypeStr=Inherit: Same as input
  Mux : Mux  Inputs=3
  Pll1 : Subsystem
  Pll2 : Subsystem
  Pll3 : Subsystem
  Sum : Sum  Inputs=|++
  delta_abc : Outport  VectorParamsAs1DForOutWhenUnconnected=off
  wires:
  Vabc_LN_pu/1 -> Demux/1
  Demux/1 -> Pll3/1(señal)
  2pi60'3/1 -> Pll3/2(w)
  Pll3/1(f cos (rad)) -> Gain1/1
  Demux/2 -> Pll1/1(señal)
  2pi60'1/1 -> Pll1/2(w)
  Gain2/1 -> Mux/2
  Demux/3 -> Pll2/1(señal)
  2pi60'2/1 -> Pll2/2(w)
  Pll2/1(f cos (rad)) -> Gain3/1
  Gain3/1 -> Mux/3
  Pll1/1(f cos (rad)) -> Gain2/1
  Mux/1 -> Sum/1
  Gain1/1 -> Mux/1
  Constant/1 -> Sum/2
  Sum/1 -> delta_abc/1

== system Model_14Bus_AC_DC_Microgrid/Bus_5/Power Factor Block1 ==
  Vabc : Inport
  Iabc : Inport  Port=2
  Complex to Magnitude-Angle : ComplexToMagnitudeAngle
  Conv pu1 : Gain  Gain=sqrt (3) /Vnom_sec  SaturateOnIntegerOverflow=on  OutDataTypeStr=Inherit: Same as input  ParamDataTypeStr=Inherit: Same as input
  Mux : Mux  Inputs=2
  Mux1 : Mux  Inputs=2
  Power : spsPowerLib/Power  Freq=Freq  Vinit=Vinit  Iinit=Iinit  Ts=Ts
  RMS3 : spsRMSLib/RMS  TrueRMS=on  Freq=60  RMSInit=0  Ts=0
  RMS4 : spsRMSLib/RMS  TrueRMS=on  Freq=60  RMSInit=0  Ts=0
  Real-Imag to Complex : RealImagToComplex
  Terminator : Terminator
  compara : Gain  SaturateOnIntegerOverflow=on  OutDataTypeStr=Inherit: Same as input  ParamDataTypeStr=Inherit: Same as input
  cos(theta) : Trigonometry  Operator=cos
  to Kw : Gain  Gain=1/1000
  to Kw1 : Gain  Gain=1/1000
  Pabc : Outport  VectorParamsAs1DForOutWhenUnconnected=off
  Qabc : Outport  Port=2  VectorParamsAs1DForOutWhenUnconnected=off
  Vabc y Vabc (rms) : Outport  Port=3  VectorParamsAs1DForOutWhenUnconnected=off
  Iabc y Iabc (rms) : Outport  Port=4  VectorParamsAs1DForOutWhenUnconnected=off
  "PFabc " : Outport  Port=5  VectorParamsAs1DForOutWhenUnconnected=off
  tag scope: P_abc_Bus5=global, Q_abc_Bus5=global, Vabc_LL_pu_Bus5=global
  wires:
  Complex to Magnitude-Angle/2 -> cos(theta)/1
  Real-Imag to Complex/1 -> Complex to Magnitude-Angle/1
  cos(theta)/1 -> "PFabc "/1
  Complex to Magnitude-Angle/1 -> Terminator/1
  Iabc/1 -> RMS4/1, compara/1, Power/2
  RMS4/1 -> Mux1/2
  Mux1/1 -> Iabc y Iabc (rms)/1
  Mux/1 -> Vabc y Vabc (rms)/1
  Vabc/1 -> Power/1, Mux/2, RMS3/1
  compara/1 -> Mux1/1
  Conv pu1/1 -> [Vabc_LL_pu_Bus5]
  RMS3/1 -> Conv pu1/1, Mux/1
  Power/2 -> Qabc/1, Real-Imag to Complex/2, to Kw/1
  Power/1 -> to Kw1/1, Pabc/1, Real-Imag to Complex/1
  to Kw/1 -> [Q_abc_Bus5]
  to Kw1/1 -> [P_abc_Bus5]

== system Model_14Bus_AC_DC_Microgrid/Bus_6 /PLL ==
  Vabc_LN_pu : Inport
  2pi60'1 : Constant  Value=2*pi*60
  2pi60'2 : Constant  Value=2*pi*60
  2pi60'3 : Constant  Value=2*pi*60
  Constant : Constant  Value=90
  Demux : Demux  Outputs=3
  Gain1 : Gain  Gain=180/pi  SaturateOnIntegerOverflow=on  OutDataTypeStr=Inherit: Same as input  ParamDataTypeStr=Inherit: Same as input
  Gain2 : Gain  Gain=180/pi  SaturateOnIntegerOverflow=on  OutDataTypeStr=Inherit: Same as input  ParamDataTypeStr=Inherit: Same as input
  Gain3 : Gain  Gain=180/pi  SaturateOnIntegerOverflow=on  OutDataTypeStr=Inherit: Same as input  ParamDataTypeStr=Inherit: Same as input
  Mux : Mux  Inputs=3
  Pll1 : Subsystem
  Pll2 : Subsystem
  Pll3 : Subsystem
  Sum : Sum  Inputs=|++
  delta_abc : Outport  VectorParamsAs1DForOutWhenUnconnected=off
  wires:
  Vabc_LN_pu/1 -> Demux/1
  Demux/1 -> Pll3/1(señal)
  2pi60'3/1 -> Pll3/2(w)
  Pll3/1(f cos (rad)) -> Gain1/1
  Demux/2 -> Pll1/1(señal)
  2pi60'1/1 -> Pll1/2(w)
  Gain2/1 -> Mux/2
  Demux/3 -> Pll2/1(señal)
  2pi60'2/1 -> Pll2/2(w)
  Pll2/1(f cos (rad)) -> Gain3/1
  Gain3/1 -> Mux/3
  Pll1/1(f cos (rad)) -> Gain2/1
  Mux/1 -> Sum/1
  Gain1/1 -> Mux/1
  Constant/1 -> Sum/2
  Sum/1 -> delta_abc/1

== system Model_14Bus_AC_DC_Microgrid/Bus_6 /Power Factor Block1 ==
  Vabc : Inport
  Iabc : Inport  Port=2
  Complex to Magnitude-Angle : ComplexToMagnitudeAngle
  Conv pu2 : Gain  Gain=sqrt (3) /Vnom_prim  SaturateOnIntegerOverflow=on  OutDataTypeStr=Inherit: Same as input  ParamDataTypeStr=Inherit: Same as input
  Mux : Mux  Inputs=2
  Mux1 : Mux  Inputs=2
  Power : spsPowerLib/Power  Freq=Freq  Vinit=Vinit  Iinit=Iinit  Ts=Ts
  RMS3 : spsRMSLib/RMS  TrueRMS=on  Freq=60  RMSInit=0  Ts=0
  RMS4 : spsRMSLib/RMS  TrueRMS=on  Freq=60  RMSInit=0  Ts=0
  Real-Imag to Complex : RealImagToComplex
  Terminator : Terminator
  compara : Gain  SaturateOnIntegerOverflow=on  OutDataTypeStr=Inherit: Same as input  ParamDataTypeStr=Inherit: Same as input
  cos(theta) : Trigonometry  Operator=cos
  to Kw : Gain  Gain=1/1000
  to Kw1 : Gain  Gain=1/1000
  Pabc : Outport  VectorParamsAs1DForOutWhenUnconnected=off
  Qabc : Outport  Port=2  VectorParamsAs1DForOutWhenUnconnected=off
  Vabc y Vabc (rms) : Outport  Port=3  VectorParamsAs1DForOutWhenUnconnected=off
  Iabc y Iabc (rms) : Outport  Port=4  VectorParamsAs1DForOutWhenUnconnected=off
  "PFabc " : Outport  Port=5  VectorParamsAs1DForOutWhenUnconnected=off
  tag scope: P_abc_Bus6=global, Q_abc_Bus6=global, Vabc_LL_pu_Bus6=global
  wires:
  Complex to Magnitude-Angle/2 -> cos(theta)/1
  Real-Imag to Complex/1 -> Complex to Magnitude-Angle/1
  cos(theta)/1 -> "PFabc "/1
  Complex to Magnitude-Angle/1 -> Terminator/1
  Iabc/1 -> RMS4/1, compara/1, Power/2
  RMS4/1 -> Mux1/2
  Mux1/1 -> Iabc y Iabc (rms)/1
  Mux/1 -> Vabc y Vabc (rms)/1
  Vabc/1 -> Power/1, Mux/2, RMS3/1
  compara/1 -> Mux1/1
  RMS3/1 -> Conv pu2/1, Mux/1
  Conv pu2/1 -> [Vabc_LL_pu_Bus6]
  Power/2 -> Qabc/1, Real-Imag to Complex/2, to Kw/1
  Power/1 -> to Kw1/1, Pabc/1, Real-Imag to Complex/1
  to Kw/1 -> [Q_abc_Bus6]
  to Kw1/1 -> [P_abc_Bus6]

== system Model_14Bus_AC_DC_Microgrid/Bus_7/PLL ==
  Vabc_LN_pu : Inport
  2pi60'1 : Constant  Value=2*pi*60
  2pi60'2 : Constant  Value=2*pi*60
  2pi60'3 : Constant  Value=2*pi*60
  Constant : Constant  Value=90
  Demux : Demux  Outputs=3
  Gain1 : Gain  Gain=180/pi  SaturateOnIntegerOverflow=on  OutDataTypeStr=Inherit: Same as input  ParamDataTypeStr=Inherit: Same as input
  Gain2 : Gain  Gain=180/pi  SaturateOnIntegerOverflow=on  OutDataTypeStr=Inherit: Same as input  ParamDataTypeStr=Inherit: Same as input
  Gain3 : Gain  Gain=180/pi  SaturateOnIntegerOverflow=on  OutDataTypeStr=Inherit: Same as input  ParamDataTypeStr=Inherit: Same as input
  Mux : Mux  Inputs=3
  Pll1 : Subsystem
  Pll2 : Subsystem
  Pll3 : Subsystem
  Sum : Sum  Inputs=|++
  delta_abc : Outport  VectorParamsAs1DForOutWhenUnconnected=off
  wires:
  Vabc_LN_pu/1 -> Demux/1
  Demux/1 -> Pll3/1(señal)
  2pi60'3/1 -> Pll3/2(w)
  Pll3/1(f cos (rad)) -> Gain1/1
  Demux/2 -> Pll1/1(señal)
  2pi60'1/1 -> Pll1/2(w)
  Gain2/1 -> Mux/2
  Demux/3 -> Pll2/1(señal)
  2pi60'2/1 -> Pll2/2(w)
  Pll2/1(f cos (rad)) -> Gain3/1
  Gain3/1 -> Mux/3
  Pll1/1(f cos (rad)) -> Gain2/1
  Mux/1 -> Sum/1
  Gain1/1 -> Mux/1
  Constant/1 -> Sum/2
  Sum/1 -> delta_abc/1

== system Model_14Bus_AC_DC_Microgrid/Bus_7/Power Factor Block1 ==
  Vabc : Inport
  Iabc : Inport  Port=2
  Complex to Magnitude-Angle : ComplexToMagnitudeAngle
  Conv pu2 : Gain  Gain=sqrt (3) /Vnom_prim  SaturateOnIntegerOverflow=on  OutDataTypeStr=Inherit: Same as input  ParamDataTypeStr=Inherit: Same as input
  Mux : Mux  Inputs=2
  Mux1 : Mux  Inputs=2
  Power : spsPowerLib/Power  Freq=Freq  Vinit=Vinit  Iinit=Iinit  Ts=Ts
  RMS3 : spsRMSLib/RMS  TrueRMS=on  Freq=60  RMSInit=0  Ts=0
  RMS4 : spsRMSLib/RMS  TrueRMS=on  Freq=60  RMSInit=0  Ts=0
  Real-Imag to Complex : RealImagToComplex
  Terminator : Terminator
  compara : Gain  SaturateOnIntegerOverflow=on  OutDataTypeStr=Inherit: Same as input  ParamDataTypeStr=Inherit: Same as input
  cos(theta) : Trigonometry  Operator=cos
  to Kw : Gain  Gain=1/1000
  to Kw1 : Gain  Gain=1/1000
  Pabc : Outport  VectorParamsAs1DForOutWhenUnconnected=off
  Qabc : Outport  Port=2  VectorParamsAs1DForOutWhenUnconnected=off
  Vabc y Vabc (rms) : Outport  Port=3  VectorParamsAs1DForOutWhenUnconnected=off
  Iabc y Iabc (rms) : Outport  Port=4  VectorParamsAs1DForOutWhenUnconnected=off
  "PFabc " : Outport  Port=5  VectorParamsAs1DForOutWhenUnconnected=off
  tag scope: P_abc_Bus7=global, Q_abc_Bus7=global, Vabc_LL_pu_Bus7=global
  wires:
  Complex to Magnitude-Angle/2 -> cos(theta)/1
  Real-Imag to Complex/1 -> Complex to Magnitude-Angle/1
  cos(theta)/1 -> "PFabc "/1
  Complex to Magnitude-Angle/1 -> Terminator/1
  Iabc/1 -> RMS4/1, compara/1, Power/2
  RMS4/1 -> Mux1/2
  Mux1/1 -> Iabc y Iabc (rms)/1
  Mux/1 -> Vabc y Vabc (rms)/1
  Vabc/1 -> Power/1, Mux/2, RMS3/1
  compara/1 -> Mux1/1
  Conv pu2/1 -> [Vabc_LL_pu_Bus7]
  RMS3/1 -> Conv pu2/1, Mux/1
  Power/2 -> Qabc/1, Real-Imag to Complex/2, to Kw/1
  Power/1 -> to Kw1/1, Pabc/1, Real-Imag to Complex/1
  to Kw/1 -> [Q_abc_Bus7]
  to Kw1/1 -> [P_abc_Bus7]

== system Model_14Bus_AC_DC_Microgrid/Bus_8      /PLL ==
  Vabc_LN_pu : Inport
  2pi60'1 : Constant  Value=2*pi*60
  2pi60'2 : Constant  Value=2*pi*60
  2pi60'3 : Constant  Value=2*pi*60
  Constant : Constant  Value=90
  Demux : Demux  Outputs=3
  Gain1 : Gain  Gain=180/pi  SaturateOnIntegerOverflow=on  OutDataTypeStr=Inherit: Same as input  ParamDataTypeStr=Inherit: Same as input
  Gain2 : Gain  Gain=180/pi  SaturateOnIntegerOverflow=on  OutDataTypeStr=Inherit: Same as input  ParamDataTypeStr=Inherit: Same as input
  Gain3 : Gain  Gain=180/pi  SaturateOnIntegerOverflow=on  OutDataTypeStr=Inherit: Same as input  ParamDataTypeStr=Inherit: Same as input
  Mux : Mux  Inputs=3
  Pll1 : Subsystem
  Pll2 : Subsystem
  Pll3 : Subsystem
  Sum : Sum  Inputs=|++
  delta_abc : Outport  VectorParamsAs1DForOutWhenUnconnected=off
  wires:
  Vabc_LN_pu/1 -> Demux/1
  Demux/1 -> Pll3/1(señal)
  2pi60'3/1 -> Pll3/2(w)
  Pll3/1(f cos (rad)) -> Gain1/1
  Demux/2 -> Pll1/1(señal)
  2pi60'1/1 -> Pll1/2(w)
  Gain2/1 -> Mux/2
  Demux/3 -> Pll2/1(señal)
  2pi60'2/1 -> Pll2/2(w)
  Pll2/1(f cos (rad)) -> Gain3/1
  Gain3/1 -> Mux/3
  Pll1/1(f cos (rad)) -> Gain2/1
  Mux/1 -> Sum/1
  Gain1/1 -> Mux/1
  Constant/1 -> Sum/2
  Sum/1 -> delta_abc/1

== system Model_14Bus_AC_DC_Microgrid/Bus_8      /Power Factor Block1 ==
  Vabc : Inport
  Iabc : Inport  Port=2
  Complex to Magnitude-Angle : ComplexToMagnitudeAngle
  Conv pu2 : Gain  Gain=sqrt (3) /Vnom_Diesel  SaturateOnIntegerOverflow=on  OutDataTypeStr=Inherit: Same as input  ParamDataTypeStr=Inherit: Same as input
  Gain : Gain  Gain=-1/1000
  Gain1 : Gain  Gain=-1/1000
  Mux : Mux  Inputs=2
  Mux1 : Mux  Inputs=2
  Power : spsPowerLib/Power  Freq=Freq  Vinit=Vinit  Iinit=Iinit  Ts=Ts
  RMS3 : spsRMSLib/RMS  TrueRMS=on  Freq=60  RMSInit=0  Ts=0
  RMS4 : spsRMSLib/RMS  TrueRMS=on  Freq=60  RMSInit=0  Ts=0
  Real-Imag to Complex : RealImagToComplex
  Terminator : Terminator
  compara : Gain  SaturateOnIntegerOverflow=on  OutDataTypeStr=Inherit: Same as input  ParamDataTypeStr=Inherit: Same as input
  cos(theta) : Trigonometry  Operator=cos
  Pabc : Outport  VectorParamsAs1DForOutWhenUnconnected=off
  Qabc : Outport  Port=2  VectorParamsAs1DForOutWhenUnconnected=off
  Vabc y Vabc (rms) : Outport  Port=3  VectorParamsAs1DForOutWhenUnconnected=off
  Iabc y Iabc (rms) : Outport  Port=4  VectorParamsAs1DForOutWhenUnconnected=off
  "PFabc " : Outport  Port=5  VectorParamsAs1DForOutWhenUnconnected=off
  tag scope: P_abc_Bus8=global, Q_abc_Bus8=global, Vabc_LL_pu_Bus8=global
  wires:
  Complex to Magnitude-Angle/2 -> cos(theta)/1
  Real-Imag to Complex/1 -> Complex to Magnitude-Angle/1
  cos(theta)/1 -> "PFabc "/1
  Complex to Magnitude-Angle/1 -> Terminator/1
  Iabc/1 -> RMS4/1, compara/1, Power/2
  RMS4/1 -> Mux1/2
  Mux1/1 -> Iabc y Iabc (rms)/1
  Mux/1 -> Vabc y Vabc (rms)/1
  Vabc/1 -> Power/1, Mux/2, RMS3/1
  compara/1 -> Mux1/1
  Conv pu2/1 -> [Vabc_LL_pu_Bus8]
  RMS3/1 -> Conv pu2/1, Mux/1
  Power/2 -> Qabc/1, Real-Imag to Complex/2, Gain/1
  Power/1 -> Gain1/1, Pabc/1, Real-Imag to Complex/1
  Gain/1 -> [Q_abc_Bus8]
  Gain1/1 -> [P_abc_Bus8]

== system Model_14Bus_AC_DC_Microgrid/Bus_9/PLL ==
  Vabc_LN_pu : Inport
  2pi60'1 : Constant  Value=2*pi*60
  2pi60'2 : Constant  Value=2*pi*60
  2pi60'3 : Constant  Value=2*pi*60
  Constant : Constant  Value=90
  Demux : Demux  Outputs=3
  Gain1 : Gain  Gain=180/pi  SaturateOnIntegerOverflow=on  OutDataTypeStr=Inherit: Same as input  ParamDataTypeStr=Inherit: Same as input
  Gain2 : Gain  Gain=180/pi  SaturateOnIntegerOverflow=on  OutDataTypeStr=Inherit: Same as input  ParamDataTypeStr=Inherit: Same as input
  Gain3 : Gain  Gain=180/pi  SaturateOnIntegerOverflow=on  OutDataTypeStr=Inherit: Same as input  ParamDataTypeStr=Inherit: Same as input
  Mux : Mux  Inputs=3
  Pll1 : Subsystem
  Pll2 : Subsystem
  Pll3 : Subsystem
  Sum : Sum  Inputs=|++
  delta_abc : Outport  VectorParamsAs1DForOutWhenUnconnected=off
  wires:
  Vabc_LN_pu/1 -> Demux/1
  Demux/1 -> Pll3/1(señal)
  2pi60'3/1 -> Pll3/2(w)
  Pll3/1(f cos (rad)) -> Gain1/1
  Demux/2 -> Pll1/1(señal)
  2pi60'1/1 -> Pll1/2(w)
  Gain2/1 -> Mux/2
  Demux/3 -> Pll2/1(señal)
  2pi60'2/1 -> Pll2/2(w)
  Pll2/1(f cos (rad)) -> Gain3/1
  Gain3/1 -> Mux/3
  Pll1/1(f cos (rad)) -> Gain2/1
  Mux/1 -> Sum/1
  Gain1/1 -> Mux/1
  Constant/1 -> Sum/2
  Sum/1 -> delta_abc/1

== system Model_14Bus_AC_DC_Microgrid/Bus_9/Power Factor Block1 ==
  Vabc : Inport
  Iabc : Inport  Port=2
  Complex to Magnitude-Angle : ComplexToMagnitudeAngle
  Conv pu2 : Gain  Gain=sqrt (3) /Vnom_prim  SaturateOnIntegerOverflow=on  OutDataTypeStr=Inherit: Same as input  ParamDataTypeStr=Inherit: Same as input
  Mux : Mux  Inputs=2
  Mux1 : Mux  Inputs=2
  Power : spsPowerLib/Power  Freq=Freq  Vinit=Vinit  Iinit=Iinit  Ts=Ts
  RMS3 : spsRMSLib/RMS  TrueRMS=on  Freq=60  RMSInit=0  Ts=0
  RMS4 : spsRMSLib/RMS  TrueRMS=on  Freq=60  RMSInit=0  Ts=0
  Real-Imag to Complex : RealImagToComplex
  Terminator : Terminator
  compara : Gain  SaturateOnIntegerOverflow=on  OutDataTypeStr=Inherit: Same as input  ParamDataTypeStr=Inherit: Same as input
  cos(theta) : Trigonometry  Operator=cos
  to Kw : Gain  Gain=1/1000
  to Kw1 : Gain  Gain=1/1000
  Pabc : Outport  VectorParamsAs1DForOutWhenUnconnected=off
  Qabc : Outport  Port=2  VectorParamsAs1DForOutWhenUnconnected=off
  Vabc y Vabc (rms) : Outport  Port=3  VectorParamsAs1DForOutWhenUnconnected=off
  Iabc y Iabc (rms) : Outport  Port=4  VectorParamsAs1DForOutWhenUnconnected=off
  "PFabc " : Outport  Port=5  VectorParamsAs1DForOutWhenUnconnected=off
  tag scope: P_abc_Bus9=global, Q_abc_Bus9=global, Vabc_LL_pu_Bus9=global
  wires:
  Complex to Magnitude-Angle/2 -> cos(theta)/1
  Real-Imag to Complex/1 -> Complex to Magnitude-Angle/1
  cos(theta)/1 -> "PFabc "/1
  Complex to Magnitude-Angle/1 -> Terminator/1
  Iabc/1 -> RMS4/1, compara/1, Power/2
  RMS4/1 -> Mux1/2
  Mux1/1 -> Iabc y Iabc (rms)/1
  Mux/1 -> Vabc y Vabc (rms)/1
  Vabc/1 -> Power/1, Mux/2, RMS3/1
  compara/1 -> Mux1/1
  RMS3/1 -> Conv pu2/1, Mux/1
  Conv pu2/1 -> [Vabc_LL_pu_Bus9]
  Power/2 -> Qabc/1, Real-Imag to Complex/2, to Kw/1
  Power/1 -> to Kw1/1, Pabc/1, Real-Imag to Complex/1
  to Kw/1 -> [Q_abc_Bus9]
  to Kw1/1 -> [P_abc_Bus9]

== system Model_14Bus_AC_DC_Microgrid/Bus_AC PV /PLL ==
  Vabc_LN_pu : Inport
  2pi60'1 : Constant  Value=2*pi*60
  2pi60'2 : Constant  Value=2*pi*60
  2pi60'3 : Constant  Value=2*pi*60
  Constant : Constant  Value=90
  Demux : Demux  Outputs=3
  Gain1 : Gain  Gain=180/pi  SaturateOnIntegerOverflow=on  OutDataTypeStr=Inherit: Same as input  ParamDataTypeStr=Inherit: Same as input
  Gain2 : Gain  Gain=180/pi  SaturateOnIntegerOverflow=on  OutDataTypeStr=Inherit: Same as input  ParamDataTypeStr=Inherit: Same as input
  Gain3 : Gain  Gain=180/pi  SaturateOnIntegerOverflow=on  OutDataTypeStr=Inherit: Same as input  ParamDataTypeStr=Inherit: Same as input
  Mux : Mux  Inputs=3
  Pll1 : Subsystem
  Pll2 : Subsystem
  Pll3 : Subsystem
  Sum : Sum  Inputs=|++
  delta_abc : Outport  VectorParamsAs1DForOutWhenUnconnected=off
  wires:
  Vabc_LN_pu/1 -> Demux/1
  Demux/1 -> Pll3/1(señal)
  2pi60'3/1 -> Pll3/2(w)
  Pll3/1(f cos (rad)) -> Gain1/1
  Demux/2 -> Pll1/1(señal)
  2pi60'1/1 -> Pll1/2(w)
  Gain2/1 -> Mux/2
  Demux/3 -> Pll2/1(señal)
  2pi60'2/1 -> Pll2/2(w)
  Pll2/1(f cos (rad)) -> Gain3/1
  Gain3/1 -> Mux/3
  Pll1/1(f cos (rad)) -> Gain2/1
  Mux/1 -> Sum/1
  Gain1/1 -> Mux/1
  Constant/1 -> Sum/2
  Sum/1 -> delta_abc/1

== system Model_14Bus_AC_DC_Microgrid/Bus_AC PV /Power Factor Block1 ==
  Vabc : Inport
  Iabc : Inport  Port=2
  Complex to Magnitude-Angle : ComplexToMagnitudeAngle
  Mux : Mux  Inputs=2
  Mux1 : Mux  Inputs=2
  Power : spsPowerLib/Power  Freq=Freq  Vinit=Vinit  Iinit=Iinit  Ts=Ts
  RMS3 : spsRMSLib/RMS  TrueRMS=on  Freq=60  RMSInit=0  Ts=0
  RMS4 : spsRMSLib/RMS  TrueRMS=on  Freq=60  RMSInit=0  Ts=0
  Real-Imag to Complex : RealImagToComplex
  Terminator : Terminator
  compara : Gain  SaturateOnIntegerOverflow=on  OutDataTypeStr=Inherit: Same as input  ParamDataTypeStr=Inherit: Same as input
  cos(theta) : Trigonometry  Operator=cos
  Pabc : Outport  VectorParamsAs1DForOutWhenUnconnected=off
  Qabc : Outport  Port=2  VectorParamsAs1DForOutWhenUnconnected=off
  Vabc y Vabc (rms) : Outport  Port=3  VectorParamsAs1DForOutWhenUnconnected=off
  Iabc y Iabc (rms) : Outport  Port=4  VectorParamsAs1DForOutWhenUnconnected=off
  "PFabc " : Outport  Port=5  VectorParamsAs1DForOutWhenUnconnected=off
  wires:
  Power/1 -> Pabc/1, Real-Imag to Complex/1
  Power/2 -> Qabc/1, Real-Imag to Complex/2
  Complex to Magnitude-Angle/2 -> cos(theta)/1
  Real-Imag to Complex/1 -> Complex to Magnitude-Angle/1
  cos(theta)/1 -> "PFabc "/1
  Complex to Magnitude-Angle/1 -> Terminator/1
  Iabc/1 -> RMS4/1, compara/1, Power/2
  RMS4/1 -> Mux1/2
  Mux1/1 -> Iabc y Iabc (rms)/1
  Mux/1 -> Vabc y Vabc (rms)/1
  Vabc/1 -> Power/1, Mux/2, RMS3/1
  compara/1 -> Mux1/1
  RMS3/1 -> Mux/1

== system Model_14Bus_AC_DC_Microgrid/Bus_AC//DC3/Battery system ==
  note: DC Bus
  note: Bettery
  "0 = Enable (Do it after transient, so that it does not calculate ripples during transient) 1 = Reset after every change in current reference" : Constant  Value=0
  Current Inst : Scope
      settings: TimeSpan=3  ActiveDisplayYMinimum=-95.69198  ActiveDisplayYMaximum=18.63726  DataLoggingVariableName=ScopeData14
  Current going to/ from the battery : Scope
      settings: TimeSpan=3  ActiveDisplayYMinimum=-16.01322  ActiveDisplayYMaximum=9.58188  DataLoggingVariableName=ScopeData18
  Display6 : Display
  Mean : spsMeanLib/Mean  Freq=10  Vinit=0  Ts=0
  Power : Product
  Power Bess : Scope
      settings: TimeSpan=3  ActiveDisplayYMinimum=-1.69927  ActiveDisplayYMaximum=8.89728  DataLoggingVariableName=ScopeData16
  Ripple Calculations : Subsystem
  Ripple in Boost : Display
  Ripple in Buck : Display
  Vbat : Scope
      settings: ActiveDisplayYMinimum=67.95036  ActiveDisplayYMaximum=146.85504  DataLoggingVariableName=ScopeData17
  Vdc : Scope
      settings: ActiveDisplayYMinimum=-33.61714  ActiveDisplayYMaximum=302.55978  DataLoggingVariableName=ScopeData15
  to Kw : Gain  Gain=1/1000
  wires:
  to Kw/1 -> Display6/1, Power Bess/1
  Mean/1 -> Power/2
  Power/1 -> to Kw/1
  Ripple Calculations/1(Ripple in Buck) -> Ripple in Buck/1
  "0 = Enable (Do it after transient, so that it does not calculate ripples during transient) 1 = Reset after every change in current reference"/1 -> Ripple Calculations/2(Reset)
  Ripple Calculations/2(Ripple in Boost) -> Ripple in Boost/1
  [Idc_bus] -> Mean/1, Ripple Calculations/1(Signal), Current Inst/1
  [current] -> Current going to/ from the battery/1
  [Vdc_bus] -> Vdc/1, Power/1
  [Vdc_battery] -> Vbat/1

== system Model_14Bus_AC_DC_Microgrid/Bus_AC//DC3/PV system ==
  note: Bus DC
  note: PV
  Bus Selector : BusSelector  OutputSignals=V_PV,I_PV,I_diode,Irradiance (W/m2),Temperature (deg C)
  Current going to/ DC bus : Scope
      settings: TimeSpan=3  ActiveDisplayYMinimum=-0.69606  ActiveDisplayYMaximum=7.97496  DataLoggingVariableName=ScopeData12
  "P (kW) " : Display
      settings: Format=bank  Decimation=2000
  PV : Scope  NumInputPorts=3
      settings: TimeSpan=2  ActiveDisplayYMinimum=-195.85509  ActiveDisplayYMaximum=264.62823  DataLoggingDecimation=100  DataLoggingSaveFormat=Array
  PV1 : Scope  NumInputPorts=5
      settings: TimeSpan=2.5  ActiveDisplayYMinimum=900  ActiveDisplayYMaximum=1100  DataLoggingDecimation=100  DataLoggingVariableName=ScopeData2  DataLoggingSaveFormat=Array
  Pmean : Subsystem
  Vdc Boost : Display
      settings: Format=bank  Decimation=2000
  Vdc DC bus : Scope
      settings: ActiveDisplayYMinimum=-31.37786  ActiveDisplayYMaximum=282.40079  DataLoggingVariableName=ScopeData13
  tag scope: I_PV=global, Idiode_PV=global, Ir=global, Temp=global, V_PV=global
  wires:
  [V_PV] -> PV/1  "V_PV"
  [I_PV] -> PV/2  "I_PV"
  [Idiode_PV] -> PV/3  "Idiode_PV"
  [m_PV] -> Bus Selector/1
  Bus Selector/1 -> [V_PV]  "<V_PV>"
  Bus Selector/2 -> [I_PV]  "<I_PV>"
  Bus Selector/4 -> [Ir]  "<Irradiance (W/m2)>"
  Bus Selector/3 -> [Idiode_PV]  "<I_diode>"
  Bus Selector/5 -> [Temp]  "<Temperature (deg C)>"
  [Temp] -> PV1/2  "Temp (deg. C)"
  [D] -> PV1/5  "Duty Cycle"
  Pmean/2(V) -> Vdc Boost/1, PV1/4  "Vmean (V)"
  [Ir] -> PV1/1  "Ir (W/m^2)"
  Pmean/1(P) -> "P (kW) "/1, PV1/3  "Pmean  (kW)"
  [I_DC_bus_PV] -> Current going to/ DC bus/1
  [V_DC_bus_PV] -> Vdc DC bus/1
